simulink model "lab08q1"  (Simulink 7.1)
settings: Solver=ode45  StartTime=0.0  StopTime=100  RelTol=1e-3
InitFcn:
  | k2 = 8.7322;
  | K1= 3.2126;
values from neighbouring files (symbols this model uses):
  k1 = rlocfind(N3, D3)    [lab09m1.m]
settings Model: Creator=ALUNO  LastModifiedBy=ALUNO

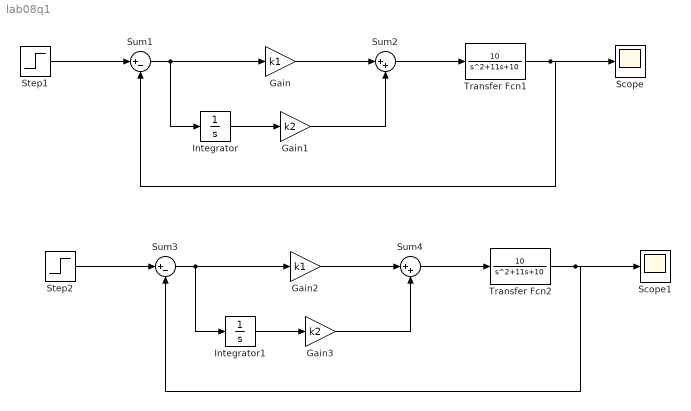
== system lab08q1 ==
  Gain : Gain  Gain=k1  ParameterDataType=sfix(16)  ParameterScaling=2^0  OutDataType=sfix(16)  OutScaling=2^0
  Gain1 : Gain  Gain=k2  ParameterDataType=sfix(16)  ParameterScaling=2^0  OutDataType=sfix(16)  OutScaling=2^0
  Gain2 : Gain  Gain=k1  ParameterDataType=sfix(16)  ParameterScaling=2^0  OutDataType=sfix(16)  OutScaling=2^0
  Gain3 : Gain  Gain=k2  ParameterDataType=sfix(16)  ParameterScaling=2^0  OutDataType=sfix(16)  OutScaling=2^0
  Integrator : Integrator
  Integrator1 : Integrator
  Scope : Scope
  Scope1 : Scope
  Step1 : Step  Time=0  SampleTime=0
  Step2 : Step  Time=0  SampleTime=0
  Sum1 : Sum  Inputs=|+-  OutDataType=sfix(16)  OutScaling=2^0
  Sum2 : Sum  Inputs=|++  OutDataType=sfix(16)  OutScaling=2^0
  Sum3 : Sum  Inputs=|+-  OutDataType=sfix(16)  OutScaling=2^0
  Sum4 : Sum  Inputs=|++  OutDataType=sfix(16)  OutScaling=2^0
  Transfer Fcn1 : TransferFcn  Numerator=[10]  Denominator=[1 11 10]
  Transfer Fcn2 : TransferFcn  Numerator=[10]  Denominator=[1 11 10]
  wires:
  Step1/1 -> Sum1/1
  Transfer Fcn1/1 -> Sum1/2, Scope/1
  Sum2/1 -> Transfer Fcn1/1
  Gain/1 -> Sum2/1
  Gain1/1 -> Sum2/2
  Integrator/1 -> Gain1/1
  Sum1/1 -> Integrator/1, Gain/1
  Step2/1 -> Sum3/1
  Transfer Fcn2/1 -> Sum3/2, Scope1/1
  Sum4/1 -> Transfer Fcn2/1
  Gain2/1 -> Sum4/1
  Gain3/1 -> Sum4/2
  Integrator1/1 -> Gain3/1
  Sum3/1 -> Integrator1/1, Gain2/1
